simulink model "PosControl_Quadruped_v3_walk"  (R2018b)
settings: Solver=FixedStepAuto  StartTime=0.0  StopTime=10  FixedStep=0.001  RelTol=1e-3  EnableMultiTasking=on
undefined symbols (not defined in the file or in its folder): robot, X, Y, Z
libraries: sm_lib x43, nesl_utility x39, Contact_Forces_Lib x4
(part 3 of 3)

== matlab function PosControl_Quadruped_v3_walk/controller/inverse kinematics3 ==
  data: x input; y input; z input; shoulder output; hip output; knee output
function [shoulder,hip,knee]= coord2theta(x,y,z)
% L1=75.0;
% L2=415.0;
% L3=408.0;


% temp = (L1*L1+L2*L2-x*x-z*z)/(2*L1*L2);
% if temp>1
%     temp = 1;
% elseif temp<-1
%     temp=1;
% end
% theta2 = pi-acos(temp);
% 
% temp = (x*x+z*z+L1*L1-L2*L2)/(2*sqrt(x*x+z*z)*L1);
% if temp>1
%     temp = 1;
% elseif temp<-1
%     temp=1;
% end
% if(x>0)
%     theta1 = abs(atan(x/z))-acos(temp);
% elseif(x<0)
%     theta1 = -abs(atan(x/z))-acos(temp);
% else
%     theta1 = -acos(temp);

L1=0;
L2=0.4;
L3=0.4;

shoulder=atan(-y/z);

%髋关节到足端长度的平方
L_H2E_2=x*x+(y-L1*sin(shoulder))*(y-L1*sin(shoulder))+(z+L1*cos(shoulder))*(z+L1*cos(shoulder));
%髋关节到足端长度
L_H2E=sqrt(L_H2E_2);

temp = (L2*L2+L_H2E_2-L3*L3)/(2*L_H2E*L2);
if temp>1
    temp = 1;
elseif temp<-1
    temp = -1;
end
Zeta=acos(temp);
hip=atan(x/(sqrt(y*y+z*z)-L1))-Zeta;

temp = (L2*L2+L3*L3-L_H2E_2)/(2*L2*L3);
if temp>1
    temp = 1;
elseif temp<-1
    temp = -1;
end
knee=pi-acos(temp);

== matlab function PosControl_Quadruped_v3_walk/controller/inverse kinematics4 ==
  data: x input; y input; z input; shoulder output; hip output; knee output
function [shoulder,hip,knee]= coord2theta(x,y,z)
% L1=75.0;
% L2=415.0;
% L3=408.0;


% temp = (L1*L1+L2*L2-x*x-z*z)/(2*L1*L2);
% if temp>1
%     temp = 1;
% elseif temp<-1
%     temp=1;
% end
% theta2 = pi-acos(temp);
% 
% temp = (x*x+z*z+L1*L1-L2*L2)/(2*sqrt(x*x+z*z)*L1);
% if temp>1
%     temp = 1;
% elseif temp<-1
%     temp=1;
% end
% if(x>0)
%     theta1 = abs(atan(x/z))-acos(temp);
% elseif(x<0)
%     theta1 = -abs(atan(x/z))-acos(temp);
% else
%     theta1 = -acos(temp);

L1=0;
L2=0.4;
L3=0.4;

shoulder=atan(-y/z);

%髋关节到足端长度的平方
L_H2E_2=x*x+(y-L1*sin(shoulder))*(y-L1*sin(shoulder))+(z+L1*cos(shoulder))*(z+L1*cos(shoulder));
%髋关节到足端长度
L_H2E=sqrt(L_H2E_2);

temp = (L2*L2+L_H2E_2-L3*L3)/(2*L_H2E*L2);
if temp>1
    temp = 1;
elseif temp<-1
    temp = -1;
end
Zeta=acos(temp);
hip=atan(x/(sqrt(y*y+z*z)-L1))-Zeta;

temp = (L2*L2+L3*L3-L_H2E_2)/(2*L2*L3);
if temp>1
    temp = 1;
elseif temp<-1
    temp = -1;
end
knee=pi-acos(temp);

== matlab function PosControl_Quadruped_v3_walk/controller/trajectory generate1 ==
  data: timer1 input; timer2 input; timer1 output; timer2 output; LegFL output; LegFR output; LegRR output; LegRL output; roll input; pitch input; yaw input; trans_x input; trans_y input; trans_z input
function [timer1,timer2,LegFL,LegFR,LegRR,LegRL] = gesture( timer1,timer2,roll,pitch,yaw,trans_x,trans_y,trans_z)

Ts = 2;

if timer2<2
    timer2 = timer2+0.001;
else
    timer1 = timer1+0.001;
    if timer1>=Ts
        timer1 = 0;
    end
end

Xs = -0.1;
Xe = 0;

Ys = 0;
Y_off = 0;

Zs = -0.55;
H = 0.15;

body_len_half = 0.35;
body_width_half = 0.2;

% O_FL = [body_len_half,body_width_half,Zs,1]';
% O_FR = [body_len_half,-body_width_half,Zs,1]';
% O_RR = [-body_len_half,-body_width_half,Zs,1]';
% O_RL = [-body_len_half,body_width_half,Zs,1]';
% 
% FL = [body_len_half,body_width_half,0]';
% FR = [body_len_half,-body_width_half,0]';
% RR = [-body_len_half,-body_width_half,0]';
% RL = [-body_len_half,body_width_half,0]';
% 
% FL_trans = [eye(3,3),FL;
%     zeros(1,3),1];
% FR_trans = [eye(3,3),FR;
%     zeros(1,3),1];
% RR_trans = [eye(3,3),RR;
%     zeros(1,3),1];
% RL_trans = [eye(3,3),RL;
%     zeros(1,3),1];
% 
%     R_roll=[1,0,0,0;
%             0,cos(roll),-sin(roll),0;
%             0,sin(roll),cos(roll),0;
%             0,0,0,1];
%     
%     R_pitch=[cos(pitch),0,sin(pitch),0;
%             0,1,0,0;
%             -sin(pitch),0,cos(pitch),0;
%             0,0,0,1];
%     
%     R_yaw=[cos(yaw),-sin(yaw),0,0;
%             sin(yaw),cos(yaw),0,0;
%             0,0,1,0;
%             0,0,0,1];
%     
%     Trans=[eye(3,3),[trans_x,trans_y,trans_z]';
%             zeros(1,3),1];
% 
%     P_FL_all = inv(FL_trans)*Trans*O_FL;
%     P_FR_all = inv(FR_trans)*Trans*O_FR;
%     P_RR_all = inv(RR_trans)*Trans*O_RR;
%     P_RL_all = inv(RL_trans)*Trans*O_RL;

%     P_FL_all = inv(FL_trans)*R_roll*R_pitch*R_yaw*Trans*O_FL;
%     P_FR_all = inv(FR_trans)*R_roll*R_pitch*R_yaw*Trans*O_FR;
%     P_RR_all = inv(RR_trans)*R_roll*R_pitch*R_yaw*Trans*O_RR;
%     P_RL_all = inv(RL_trans)*R_roll*R_pitch*R_yaw*Trans*O_RL;
% 
% 
%     LegFL = P_FL_all(1:3)';
%     LegFR = P_FR_all(1:3)';
%     LegRR = P_RR_all(1:3)';
%     LegRL = P_RL_all(1:3)';

if timer1>=0 && timer1<=0.25*Ts %1/4周期
        
    body_move = -(timer1)/(0.25*Ts)*0.25*(Xe-Xs);
    trans_x = body_move;
    
    
    O_FL = [body_len_half+Xs,body_width_half-Ys-Y_off,Zs,1]';
    O_FR = [body_len_half+Xs,-body_width_half+Ys+Y_off,Zs,1]';
    O_RR = [-body_len_half+Xs,-body_width_half+Ys,Zs,1]';
    O_RL = [-body_len_half+Xs,body_width_half-Ys,Zs,1]';

    FL = [body_len_half,body_width_half,0]';
    FR = [body_len_half,-body_width_half,0]';
    RR = [-body_len_half,-body_width_half,0]';
    RL = [-body_len_half,body_width_half,0]';

    FL_trans = [eye(3,3),FL;
        zeros(1,3),1];
    FR_trans = [eye(3,3),FR;
        zeros(1,3),1];
    RR_trans = [eye(3,3),RR;
        zeros(1,3),1];
    RL_trans = [eye(3,3),RL;
        zeros(1,3),1];
    
    Trans=[eye(3,3),[trans_x,trans_y,trans_z]';
            zeros(1,3),1];

    P_FL_all = inv(FL_trans)*Trans*O_FL;
    P_FR_all = inv(FR_trans)*Trans*O_FR;
    P_RR_all = inv(RR_trans)*Trans*O_RR;
    P_RL_all = inv(RL_trans)*Trans*O_RL;
    
%     sigma = 2*pi*(timer1-0.4*Ts)/(0.2*Ts);
%     
%     x_f = (Xe-Xs)*((sigma-sin(sigma))/(2*pi))+Xs;  
%     z_up = H*(1-cos(sigma))/2+Zs;
    
    
    sigma = 2*pi*timer1/(0.25*Ts);

    x_f = 0.75*(Xe-Xs)*((sigma-sin(sigma))/(2*pi))+Xs;  
    z_up = H*(1-cos(sigma))/2+Zs;
    
    LegFL = [x_f,-Ys-Y_off,z_up]';
    LegFR = P_FR_all(1:3);
    LegRR = P_RR_all(1:3);
    LegRL = P_RL_all(1:3);

elseif timer1>=0.25*Ts && timer1<=0.5*Ts %2/4周期
    
    body_move = -(timer1-0.25*Ts)/(0.25*Ts)*0.25*(Xe-Xs);
    trans_x = body_move;
    
    
    O_FL = [body_len_half+Xs+0.75*(Xe-Xs),body_width_half-Ys-Y_off,Zs,1]';
    O_FR = [body_len_half+Xs-0.25*(Xe-Xs),-body_width_half+Ys+Y_off,Zs,1]';
    O_RR = [-body_len_half+Xs-0.25*(Xe-Xs),-body_width_half+Ys,Zs,1]';
    O_RL = [-body_len_half+Xs-0.25*(Xe-Xs),body_width_half-Ys,Zs,1]';

    FL = [body_len_half,body_width_half,0]';
    FR = [body_len_half,-body_width_half,0]';
    RR = [-body_len_half,-body_width_half,0]';
    RL = [-body_len_half,body_width_half,0]';

    FL_trans = [eye(3,3),FL;
        zeros(1,3),1];
    FR_trans = [eye(3,3),FR;
        zeros(1,3),1];
    RR_trans = [eye(3,3),RR;
        zeros(1,3),1];
    RL_trans = [eye(3,3),RL;
        zeros(1,3),1];
    
    Trans=[eye(3,3),[trans_x,trans_y,trans_z]';
            zeros(1,3),1];

    P_FL_all = inv(FL_trans)*Trans*O_FL;
    P_FR_all = inv(FR_trans)*Trans*O_FR;
    P_RR_all = inv(RR_trans)*Trans*O_RR;
    P_RL_all = inv(RL_trans)*Trans*O_RL;
    
    
    sigma = 2*pi*(timer1-0.25*Ts)/(0.25*Ts);
    
    x_f = 0.75*(Xe-Xs)*((sigma-sin(sigma))/(2*pi))+Xs-0.25*(Xe-Xs);  
    z_up = H*(1-cos(sigma))/2+Zs;
    
    LegFL = P_FL_all(1:3);
    LegFR = P_FR_all(1:3);
    LegRR = [x_f,Ys,z_up]';
    LegRL = P_RL_all(1:3);

elseif timer1>=0.5*Ts && timer1<=0.75*Ts %3/4周期
    body_move = -(timer1-0.5*Ts)/(0.25*Ts)*0.25*(Xe-Xs);
    trans_x = body_move;
    
    
    O_FL = [body_len_half+Xs+0.5*(Xe-Xs),body_width_half-Ys-Y_off,Zs,1]';
    O_FR = [body_len_half+Xs-0.5*(Xe-Xs),-body_width_half+Ys+Y_off,Zs,1]';
    O_RR = [-body_len_half+Xs+0.5*(Xe-Xs),-body_width_half+Ys,Zs,1]';
    O_RL = [-body_len_half+Xs-0.5*(Xe-Xs),body_width_half-Ys,Zs,1]';

    FL = [body_len_half,body_width_half,0]';
    FR = [body_len_half,-body_width_half,0]';
    RR = [-body_len_half,-body_width_half,0]';
    RL = [-body_len_half,body_width_half,0]';

    FL_trans = [eye(3,3),FL;
        zeros(1,3),1];
    FR_trans = [eye(3,3),FR;
        zeros(1,3),1];
    RR_trans = [eye(3,3),RR;
        zeros(1,3),1];
    RL_trans = [eye(3,3),RL;
        zeros(1,3),1];
    
    Trans=[eye(3,3),[trans_x,trans_y,trans_z]';
            zeros(1,3),1];

    P_FL_all = inv(FL_trans)*Trans*O_FL;
    P_FR_all = inv(FR_trans)*Trans*O_FR;
    P_RR_all = inv(RR_trans)*Trans*O_RR;
    P_RL_all = inv(RL_trans)*Trans*O_RL;
    
    
    sigma = 2*pi*(timer1-0.5*Ts)/(0.25*Ts);
    
    x_f = (Xe-Xs)*((sigma-sin(sigma))/(2*pi))+Xs-0.5*(Xe-Xs);  
    z_up = H*(1-cos(sigma))/2+Zs;
    
    LegFL = P_FL_all(1:3);
    LegFR = [x_f,Ys+Y_off,z_up]';
    LegRR = P_RR_all(1:3);
    LegRL = P_RL_all(1:3);
    
elseif timer1>=0.75*Ts && timer1<=Ts %4/4周期
    
    body_move = -(timer1-0.75*Ts)/(0.25*Ts)*0.25*(Xe-Xs);
    trans_x = body_move;
    
    
    O_FL = [body_len_half+Xs+0.25*(Xe-Xs),body_width_half-Ys-Y_off,Zs,1]';
    O_FR = [body_len_half+Xs+0.25*(Xe-Xs),-body_width_half+Ys+Y_off,Zs,1]';
    O_RR = [-body_len_half+Xs+0.25*(Xe-Xs),-body_width_half+Ys,Zs,1]';
    O_RL = [-body_len_half+Xs-0.75*(Xe-Xs),body_width_half-Ys,Zs,1]';

    FL = [body_len_half,body_width_half,0]';
    FR = [body_len_half,-body_width_half,0]';
    RR = [-body_len_half,-body_width_half,0]';
    RL = [-body_len_half,body_width_half,0]';

    FL_trans = [eye(3,3),FL;
        zeros(1,3),1];
    FR_trans = [eye(3,3),FR;
        zeros(1,3),1];
    RR_trans = [eye(3,3),RR;
        zeros(1,3),1];
    RL_trans = [eye(3,3),RL;
        zeros(1,3),1];
    
    Trans=[eye(3,3),[trans_x,trans_y,trans_z]';
            zeros(1,3),1];

    P_FL_all = inv(FL_trans)*Trans*O_FL;
    P_FR_all = inv(FR_trans)*Trans*O_FR;
    P_RR_all = inv(RR_trans)*Trans*O_RR;
    P_RL_all = inv(RL_trans)*Trans*O_RL;
    
    
    sigma = 2*pi*(timer1-0.75*Ts)/(0.25*Ts);
    
    x_f = (Xe-Xs)*((sigma-sin(sigma))/(2*pi))+Xs-0.75*(Xe-Xs);  
    z_up = H*(1-cos(sigma))/2+Zs;
    
    LegFL = P_FL_all(1:3);
    LegFR = P_FR_all(1:3);
    LegRR = P_RR_all(1:3);
    LegRL = [x_f,-Ys,z_up]';
    
else
    LegFL = [Xs,-Ys-Y_off,Zs]';
    LegFR = [Xs,Ys+Y_off,Zs]';
    LegRR = [Xs,Ys,Zs]';
    LegRL = [Xs,-Ys,Zs]';
end

== matlab function PosControl_Quadruped_v3_walk/controller/inverse kinematics2 ==
  data: x input; y input; z input; shoulder output; hip output; knee output
function [shoulder,hip,knee]= coord2theta(x,y,z)
% L1=75.0;
% L2=415.0;
% L3=408.0;


% temp = (L1*L1+L2*L2-x*x-z*z)/(2*L1*L2);
% if temp>1
%     temp = 1;
% elseif temp<-1
%     temp=1;
% end
% theta2 = pi-acos(temp);
% 
% temp = (x*x+z*z+L1*L1-L2*L2)/(2*sqrt(x*x+z*z)*L1);
% if temp>1
%     temp = 1;
% elseif temp<-1
%     temp=1;
% end
% if(x>0)
%     theta1 = abs(atan(x/z))-acos(temp);
% elseif(x<0)
%     theta1 = -abs(atan(x/z))-acos(temp);
% else
%     theta1 = -acos(temp);

L1=0;
L2=0.4;
L3=0.4;

shoulder=atan(-y/z);

%髋关节到足端长度的平方
L_H2E_2=x*x+(y-L1*sin(shoulder))*(y-L1*sin(shoulder))+(z+L1*cos(shoulder))*(z+L1*cos(shoulder));
%髋关节到足端长度
L_H2E=sqrt(L_H2E_2);

temp = (L2*L2+L_H2E_2-L3*L3)/(2*L_H2E*L2);
if temp>1
    temp = 1;
elseif temp<-1
    temp = -1;
end
Zeta=acos(temp);
hip=atan(x/(sqrt(y*y+z*z)-L1))-Zeta;

temp = (L2*L2+L3*L3-L_H2E_2)/(2*L2*L3);
if temp>1
    temp = 1;
elseif temp<-1
    temp = -1;
end
knee=pi-acos(temp);
